simulink library "CEO"  (R2016a)
settings: Solver=ode45  StartTime=0.0  StopTime=10.0  RelTol=1e-3
libraries: CEO x2
settings Model: Creator=rconan  LastModifiedBy=rconan
settings DataIOCC: LimitDataPoints=on
settings DebuggingCC: AllowSymbolicDim=off

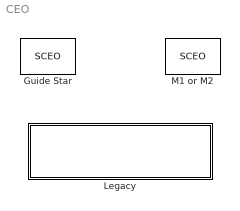
== system CEO ==
  Guide Star : M-S-Function  FunctionName=SCEO  mask(OpticalPath){source_prm=struct('data',[]), sensor=GeometricShackHartmann, sensor_prm=struct('data',[]), sensor_calib=struct('calibrations',[],'filename',[],'pseudo_inverse',[]), sensor_out=[], sampleTime=[1,0]}
      mask prompts: source_prm "Parameters"; sensor "Type"; sensor_prm "Parameters"; sensor_calib "Calibration"; sensor_out "Outputs"; sampleTime "Sample Time"
      mask help: Generate a Guide Star and an optional optical sensor
      mask init:
      | class_id = 'OP';
      | msg_box = ceo.dealer(class_id,get_param(gcb,'Name'));
      | set(gcbh,'UserData',msg_box)
      | mask = Simulink.Mask.get(gcb);
      | n_in = 2;
      | dims_in = [];
      | msg_box.n_in = n_in;
      | msg_box.n_in_ceo = 0;
      | msg_box.dims_in = {1,1};
      | n_out = 0;
      | dims_out = {};
      | msg_box.sampleTime = sampleTime;
      | %% START
      | % Source
      | source_args = ceo.liftprm(source_prm);
      | % Sensor
      | prm = mask.getParameter('sensor');
      | sensor_class = prm.TypeOptions{sensor};
      | sensor_args = ceo.liftprm(sensor_prm);
      | miscellaneous_args = [];
      | calib_src_args = [];
      | start_args = struct('source_args',source_args,...
      |               'sensor_class',sensor_class,...
      |               'sensor_args',sensor_args,...
      |               'calibration_source_args',calib_src_args,...
      |               'miscellaneous_args',miscellaneous_args);
      | msg_box.start.args = start_args;
      | %% UPDATE
      | update_args = struct('inputs',[]);
      | msg_box.update.args = update_args;
      | %% OUTPUTS
      | if isempty(sensor_out)
      |     outputs_args = struct('outputs',{[]});
      | else
      |     outputs_args = struct('outputs',{cellfun(@(x) x(1) , sensor_out)} );
      |     dims_out = cellfun(@(x) x(2) , sensor_out );
      |     n_out = numel(dims_out);
      | end
      | msg_box.n_out = n_out;
      | msg_box.dims_out = dims_out;
      | msg_box.outputs.args = outputs_args;
      | %% INITIALIZECONDITIONS
      | init_args = ceo.liftprm(sensor_calib);
      | msg_box.init.args = init_args;
      | 
      | dump(msg_box)
      mask Help: web(fullfile(fileparts(which('SCEO')),'masks',[get_param(gcb,'MaskType'),'.html']))
      mask TypeOptions sensor: None | Imaging | ShackHartmann | GeometricShackHartmann | GeometricTT7
      mask DialogControl DescGroupVar Prompt: Optical Path
      mask DialogControl DescTextVar Prompt: An optical path through the telescope consists in a star and a sensor. Ray tracing is performed from the star to the exist pupil of the GMT. From the exist pupil, the wavefront of the star is Fourier propagated to the detector plane of the sensor.
      mask DialogControl Container14 Prompt: Source
      mask DialogControl Container18 Prompt: Sensor
      mask Display: fprintf('Optical\nPath')
  "Legacy " : Subsystem
  M1 or M2 : M-S-Function  FunctionName=SCEO  mask(GMTMirror){mirror=M2, TxyzRxyz=on, mode_coefs=off, n_mode=66, sampleTime=[-1,0]}
      mask prompts: TxyzRxyz "Txyz and Rxyz rigid body"; mode_coefs "Mirror mode coefficients"; sampleTime "Sample Time"
      mask help: The GMT M1 or M2 model
      mask init:
      | class_id = 'GMT';
      | msg_box = ceo.dealer(class_id,get_param(gcb,'Name'));
      | set(gcbh,'UserData',msg_box)
      | mask = Simulink.Mask.get(gcb);
      | n_in = 2;
      | msg_box.sampleTime = sampleTime;
      | 
      | gmt_mirror = get_param(gcb,'mirror');
      | 
      | %% START
      | if strcmp(gmt_mirror,'M1')
      |     mirror_args = struct(...
      |         'mirror_modes','bending modes',...
      |         'N_MODE',n_mode);
      |     dims_in = {[7,6],[7,n_mode]};
      | else
      |     mirror_args = struct(...
      |         'mirror_modes','Karhunen-Loeve',...
      |         'N_MODE',n_mode);
      |     dims_in = {[7,6],[7,n_mode]};
      | end
      | start_args = struct('mirror',gmt_mirror,'mirror_args',mirror_args);
      | msg_box.start.args = start_args;
      |          
      | %% UPDATE
      | n_in = 0;
      | inputs_args = struct();
      | update_args = struct('mirror',gmt_mirror,'inputs_args',inputs_args);
      | if TxyzRxyz
      |     n_in = n_in + 1;
      |     dims_in{n_in} = [7,6];
      |     update_args.inputs_args.('TxyzRxyz') = [];
      | end
      | if mode_coefs
      |     n_in = n_in + 1;
      |     dims_in{n_in} = [7,n_mode];
      |     update_args.inputs_args.('mode_coefs') = [];
      | end
      | msg_box.n_in = n_in;
      | msg_box.n_in_ceo = n_in;
      | msg_box.dims_in = dims_in;
      | msg_box.update.args = update_args;
      | 
      | %% OUTPUTS
      | msg_box.n_out = 0;
      | msg_box.dims_out = [];
      mask Help: web(fullfile(fileparts(which('SCEO')),'masks',[get_param(gcb,'MaskType'),'.html']))
      mask TypeOptions mirror: M1 | M2
      mask DialogControl DescGroupVar Prompt: GMT M1 or M2 segmented mirror
      mask DialogControl DescTextVar Prompt: Select to command either M1 or M2 degrees of freedom
      mask DialogControl mirror_commnand Prompt: Mirror commands
      mask Display: fprintf('GMT\nMirror')

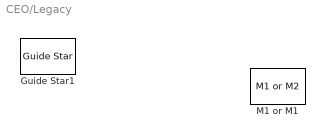
== system CEO/Legacy  ==
  Guide Star1 : CEO/Guide Star  source_prm_file='JSON/AcO_Ctrl/AcO_TT7_GUIDE_STAR.ubj'  sensor=GeometricShackHartmann  sensor_prm_file='JSON/AcO_Ctrl/AcO_TT7.ubj'  sensor_calib=struct('calibrations',[],'filename',[],'pseudo_inverse',[])  sensor_out=[]  sampleTime=[1,0]
  M1 or M1 : CEO/M1 or M2  mirror=M2  TxyzRxyz=on  mode_coefs=off  n_mode=66  sampleTime=[-1,0]
  wires:
  ? -> ?
  ? -> ?
